simulink model "qint_tt"  (Simulink 7.4)
settings: Solver=ode45  StartTime=0.0  StopTime=30  RelTol=1e-3
libraries: truetime x3
settings Model: Creator=jporter  LastModifiedBy=jporter  SimulationMode=accelerator

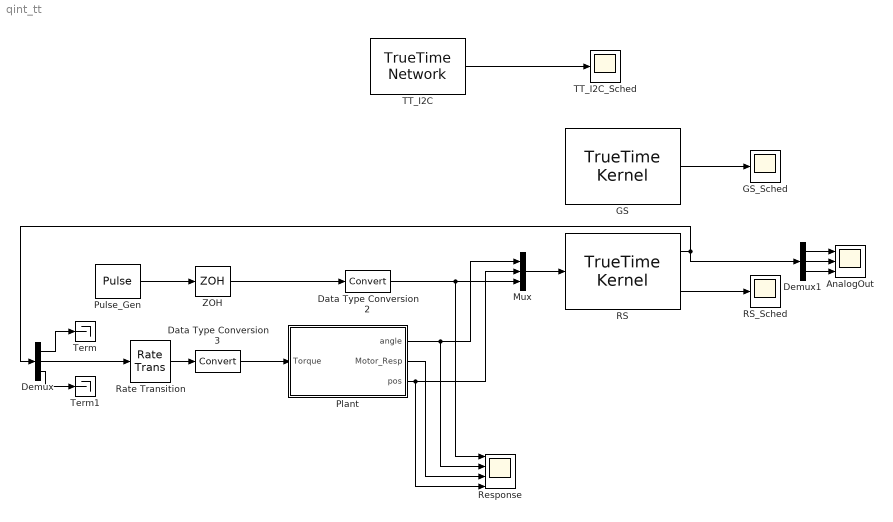
== system qint_tt ==
  AnalogOut : Scope  NumInputPorts=3
      settings: YMin=-0.8~-0.25~-1.25  YMax=0.3~0.2~1  SaveName=ScopeData2  MaxDataPoints=100000  SampleInput=on  SampleTime=0.02
  Data Type Conversion2 : DataTypeConversion
  Data Type Conversion3 : DataTypeConversion
  Demux : Demux  Outputs=3
  Demux1 : Demux  Outputs=3
  GS : truetime/TrueTime Kernel  SystemSampleTime=-1  sfun=GS_init  args=[1]  ninputsoutputs=[0 0]  ntriggers=0  trigtype=falling  nwnodenbr=[1 1]  clockoffsetdrift=[0 0]  schedoutput=on  battery=off  poweroutput=off  label=1: 1
  GS_Sched : Scope
  Mux : Mux  Inputs=3
  Plant : Subsystem
  Pulse_Gen : DiscretePulseGenerator  PulseType=Time based  Amplitude=1023  Period=10  PulseWidth=50  PhaseDelay=0  SampleTime=1
  RS : truetime/TrueTime Kernel  SystemSampleTime=-1  sfun=RS_init  args=[1]  ninputsoutputs=[3 3]  ntriggers=0  trigtype=falling  nwnodenbr=[1 2]  clockoffsetdrift=[0 0]  schedoutput=on  battery=off  poweroutput=off  label=1: 2
  RS_Sched : Scope
  Rate Transition : RateTransition
  Response : Scope  NumInputPorts=4
      settings: YMin=-5~-5~-5~-5  YMax=5~5~5~5  MaxDataPoints=100000  SampleInput=on  SampleTime=0.02
  TT_I2C : truetime/TrueTime Network  SystemSampleTime=-1  nwtype=TDMA  nwnbr=1  nnodes=2  rate=100000  minsize=512  lossprob=0  seed=0  bandwidths=[0.5 0.5]  slotsize=512  schedule=[ 1 2 ]  memsize=80000  buftype=Common buffer  overflow=Retransmit  dynSchedule=0  miniSlotSize=0  NIT=0  QSortMode=FIFO  sync=0  irtSchedule=0  nrtLength=0  nodeGraph=0  scheduleoutput=on
  TT_I2C_Sched : Scope
  Term : Terminator
  Term1 : Terminator
  ZOH : ZeroOrderHold  SampleTime=0.02
  wires:
  TT_I2C/1 -> TT_I2C_Sched/1
  GS/1 -> GS_Sched/1
  RS/2 -> RS_Sched/1
  Mux/1 -> RS/1
  Rate Transition/1 -> Data Type Conversion3/1
  Data Type Conversion3/1 -> Plant/1(Torque)
  Demux/1 -> Term/1
  Demux/3 -> Term1/1
  Pulse_Gen/1 -> ZOH/1
  Data Type Conversion2/1 -> Mux/3, Response/1
  Plant/1(angle) -> Mux/1, Response/2
  Plant/3(pos) -> Mux/2, Response/4
  ZOH/1 -> Data Type Conversion2/1
  Plant/2(Motor_Resp) -> Response/3
  Demux/2 -> Rate Transition/1
  RS/1 -> Demux/1, Demux1/1
  Demux1/1 -> AnalogOut/1
  Demux1/2 -> AnalogOut/2
  Demux1/3 -> AnalogOut/3

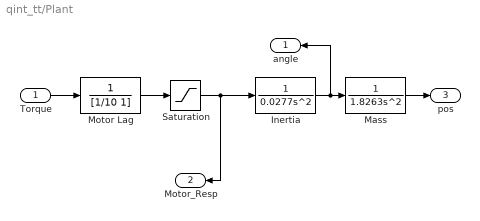
== system qint_tt/Plant ==
  Torque : Inport
  Inertia : TransferFcn  Denominator=[0.0277 0 0]
  Mass : TransferFcn  Denominator=[1.8263 0 0]
  Motor Lag : TransferFcn  Denominator=[1/10 1]
  Saturation : Saturate  UpperLimit=40  LowerLimit=-40
  angle : Outport
  Motor_Resp : Outport  Port=2
  pos : Outport  Port=3
  wires:
  Torque/1 -> Motor Lag/1
  Mass/1 -> pos/1
  Inertia/1 -> angle/1, Mass/1
  Saturation/1 -> Motor_Resp/1, Inertia/1
  Motor Lag/1 -> Saturation/1
